simulink library "filteredPIDControllerAWGS_ul"  (R2020a)
settings: Solver=VariableStepAuto  StartTime=0.0  StopTime=10.0  RelTol=1e-3
undefined symbols (not defined in the file): LaRCtrl
settings Model: Creator=mcobb  LastModifiedBy=John Jr
settings DataIOCC: ReturnWorkspaceOutputs=off
settings DebuggingCC: ArithmeticOperatorsInVariantConditions=warning
settings SFSimCC: CustomCodeUndefinedFunction=UseInterfaceOnly

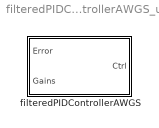
== system filteredPIDControllerAWGS_ul ==
  filteredPIDControllerAWGS : Subsystem  mask{cmax=LaRCtrl.controlSigMax.upperLimit.Value, cmin=LaRCtrl.controlSigMax.lowerLimit.Value}
      mask prompts: cmax "Control Upper Limit"; cmin "Control Lower Limit"

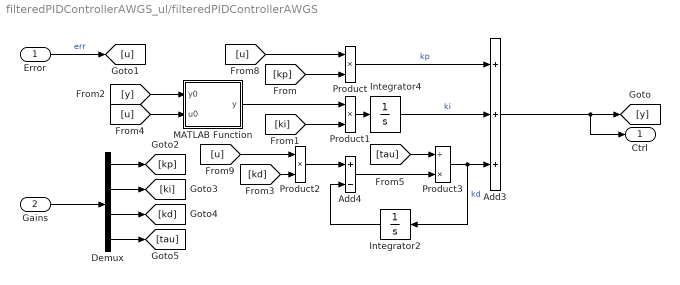
== system filteredPIDControllerAWGS_ul/filteredPIDControllerAWGS ==
  Error : Inport  PortDimensions=1
  Gains : Inport  Port=2
  Add3 : Sum  Inputs=+++
  Add4 : Sum  Inputs=+-
  Demux : Demux
  Integrator2 : Integrator
  Integrator4 : Integrator
  MATLAB Function : MATLAB Function  TreatAsAtomicUnit=on  mask{cMax=cmax, cMin=cmin}
      mask prompts: cMax "Max control value:"; cMin "Min control value:"
  Product : Product
  Product1 : Product
  Product2 : Product
  Product3 : Product  Inputs=/*
  Ctrl : Outport  PortDimensions=1  VectorParamsAs1DForOutWhenUnconnected=off
  wires:
  Demux/4 -> [tau]
  Demux/3 -> [kd]
  Demux/2 -> [ki]
  Demux/1 -> [kp]
  [u] -> MATLAB Function/2(u0)
  [y] -> MATLAB Function/1(y0)
  Error/1 -> [u]  "err"
  Integrator2/1 -> Add4/2
  Integrator4/1 -> Add3/2  "ki"
  Add3/1 -> Ctrl/1, [y]
  Product/1 -> Add3/1  "kp"
  [u] -> Product/1
  [kp] -> Product/2
  Product1/1 -> Integrator4/1
  Product2/1 -> Add4/1
  MATLAB Function/1(y) -> Product1/1
  [ki] -> Product1/2
  Product3/1 -> Integrator2/1, Add3/3  "kd"
  Add4/1 -> Product3/2
  [u] -> Product2/1
  [kd] -> Product2/2
  [tau] -> Product3/1
  Gains/1 -> Demux/1

== matlab function filteredPIDControllerAWGS_ul/filteredPIDControllerAWGS/MATLAB Function ==
  data: y0 input; u0 input; y output; cMax parameter; cMin parameter
function y = fcn(y0, u0, cMax, cMin)

if y0 > cMax
    y1 = cMax; 
elseif y0 < cMin
    y1 = cMin; 
else
    y1 = y0; 
end

sat = y0-y1; 
aw = exp(-1e5*sat^2); 
y = aw*u0;
